simulink model "RadarAltimeterFreqDomain"  (R2020b)
settings: Solver=FixedStepAuto  StartTime=0.0  StopTime=1  FixedStep=0.0000001  RelTol=1e-3
settings Model: Creator=Joseph  LastModifiedBy=Joseph

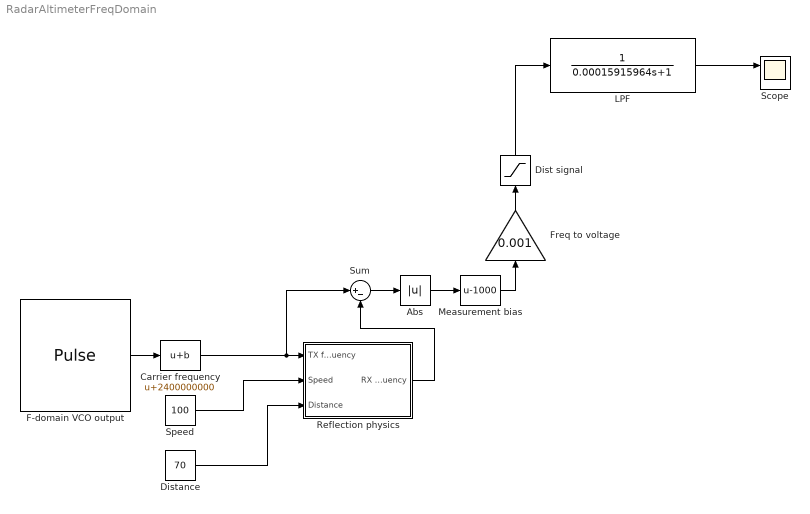
== system RadarAltimeterFreqDomain ==
  Abs : Abs
  Carrier frequency : Bias  Bias=2400000000
  Dist signal : Saturate  UpperLimit=5  LowerLimit=0
  Distance : Constant  Value=70
  F-domain VCO output : DiscretePulseGenerator  PulseType=Time based  Amplitude=10000  Period=1/125000  PulseWidth=50
  Freq to voltage : Gain  Gain=0.001
  LPF : TransferFcn  Denominator=[0.00015915964,1]
  Measurement bias : Bias  Bias=-1000
  Reflection physics : Subsystem
  Scope : Scope  NumInputPorts=2
  Speed : Constant  Value=100
  Sum : Sum  Inputs=|+-
  wires:
  F-domain VCO output/1 -> Carrier frequency/1
  Carrier frequency/1 -> Sum/1, Reflection physics/1(TX frequency)
  Reflection physics/1(RX frequency) -> Sum/2
  Speed/1 -> Reflection physics/2(Speed)
  Distance/1 -> Reflection physics/3(Distance)
  Sum/1 -> Abs/1
  Abs/1 -> Measurement bias/1
  Freq to voltage/1 -> Dist signal/1
  Dist signal/1 -> LPF/1
  LPF/1 -> Scope/1
  Measurement bias/1 -> Freq to voltage/1

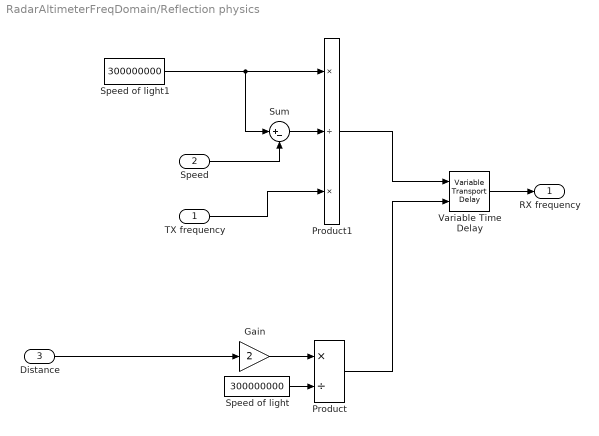
== system RadarAltimeterFreqDomain/Reflection physics ==
  TX frequency : Inport
  Speed : Inport  Port=2
  Distance : Inport  Port=3
  Gain : Gain  Gain=2
  Product : Product  Inputs=*/
  Product1 : Product  Inputs=*/*
  Speed of light : Constant  Value=300000000
  Speed of light1 : Constant  Value=300000000
  Sum : Sum  Inputs=|+-
  Variable Time Delay : VariableTransportDelay  MaximumDelay=10  InitialOutput=2.4e9
  RX frequency : Outport
  wires:
  TX frequency/1 -> Product1/3
  Gain/1 -> Product/1
  Distance/1 -> Gain/1
  Speed of light/1 -> Product/2
  Sum/1 -> Product1/2
  Speed of light1/1 -> Sum/1, Product1/1
  Variable Time Delay/1 -> RX frequency/1
  Product/1 -> Variable Time Delay/2
  Product1/1 -> Variable Time Delay/1
  Speed/1 -> Sum/2
